simulink model "example_RadiatorAIVtoEN442"  (Simulink 7.6)
settings: Solver=ode45  StartTime=0.0  StopTime=8*3600  RelTol=1e-3
undefined symbols (not defined in the file): A, B, C, Dd
libraries: carnot x9, simulink x1
settings Model: Creator=drhf  LastModifiedBy=drhf
settings CodeAppCC: CustomSymbolStrType=$N$R$M_T

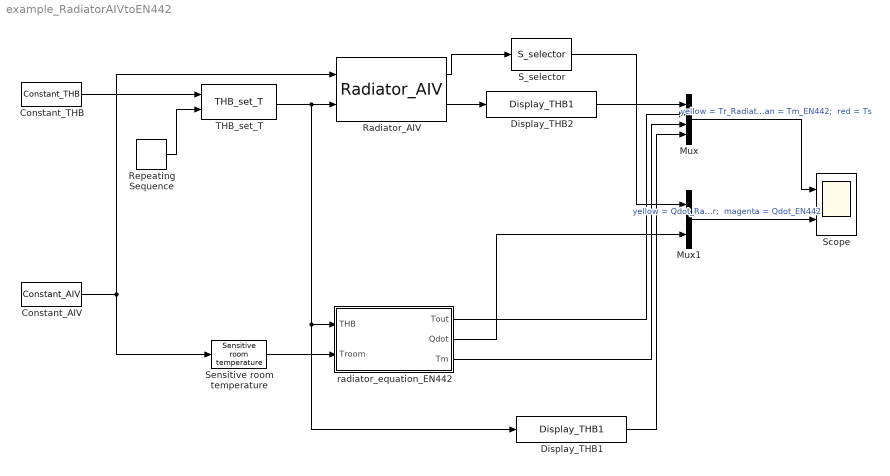
== system example_RadiatorAIVtoEN442 ==
  Constant_AIV : carnot/Source/Ventilation/Constant_AIV  SystemSampleTime=-1  Tsens=20  Tcon=20  Trad=20  mw=0.012  mco=0.01  rhoair=1.2  cpair=1004  pair=100000  nair=0.5
  Constant_THB : carnot/Source/Simple/Constant_THB  SystemSampleTime=-1  t=40  mdot=1000/4182/10  p=1e5  mID=No Pressure Drop  fluid=Water (Constant 20°C)  mix=0  dia=0.02  hgt=0
  Display_THB1 : carnot/Outputs/Display_THB1  SystemSampleTime=-1  t=on  m=off  p=off  id=off  mix=off  d=off
  Display_THB2 : carnot/Outputs/Display_THB1  SystemSampleTime=-1  t=on  m=off  p=off  id=off  mix=off  d=off
  Mux : Mux
  Mux1 : Mux  Inputs=2
  Radiator_AIV : carnot/Source/Heat_Exchanger/Radiator_AIV  SystemSampleTime=-1  pnom=1000  dtnom=50  expo=1.3  mcap=5*4182  ra=0.47  tini=20  lin=10  qua=10
  Repeating Sequence : simulink/Sources/Repeating Sequence  SystemSampleTime=-1  rep_seq_t=[0 2 2.1 4 4.1 6 6.1 8]*3600  rep_seq_y=[45 45 55 55 65 65 75 75]
  S_selector : carnot/Outputs/S_selector  SystemSampleTime=-1  e1=off  e2=off  e3=off  e4=off  e5=on  e6=off  e7=off  e8=off  e9=off  e10=off  e11=off  e12=off  e13=off
  Scope : Scope  NumInputPorts=2
      settings: YMin=-5~-5  YMax=5~5
  Sensitive room temperature : carnot/Outputs/Sensitive room temperature  SystemSampleTime=-1  share_c=47
  THB_set_T : carnot/Source/Simple/THB_set_T  SystemSampleTime=-1
  radiator_equation_EN442 : Subsystem  mask(radiator equation){pnom=1000, dtnom=50, expo=1.3, mcap=10*4200}
      mask prompts: pnom "Qdot_nom: nominal power per in W"; dtnom "Tdiff_nom: nominal temperature difference in K"; expo "radiator exponent (> 0)"; mcap "mass * capacity per unit in J/K"
      mask help:
      | The block calculates the heat transfer of a radiator to a room according to the EN 442 equation:
      | Qdot = Qdot_nom * (Tdiff/Tdiff_nom)^exponent
      | The thermal capacity of the radiator is modeled by a 1-node capacity.
      | mcp*dT/dt = mdot*cp*(Tin-Tnode)-Qdot
  wires:
  Constant_THB/1 -> THB_set_T/1
  THB_set_T/1 -> radiator_equation_EN442/1(THB), Display_THB1/1, Radiator_AIV/2
  Mux/1 -> Scope/1  "yellow = Tr_Radiator;  magenta = Tr_EN442;  cyan = Tm_EN442;  red = Ts"
  Radiator_AIV/2 -> Display_THB2/1
  Repeating Sequence/1 -> THB_set_T/2
  Display_THB2/1 -> Mux/1
  radiator_equation_EN442/1(Tout) -> Mux/2
  S_selector/1 -> Mux1/1
  radiator_equation_EN442/2(Qdot) -> Mux1/2
  Mux1/1 -> Scope/2  "yellow = Qdot_Radiator;  magenta = Qdot_EN442"
  radiator_equation_EN442/3(Tm) -> Mux/3
  Display_THB1/1 -> Mux/4
  Radiator_AIV/1 -> S_selector/1
  Sensitive room temperature/1 -> radiator_equation_EN442/2(Troom)
  Constant_AIV/1 -> Sensitive room temperature/1, Radiator_AIV/1

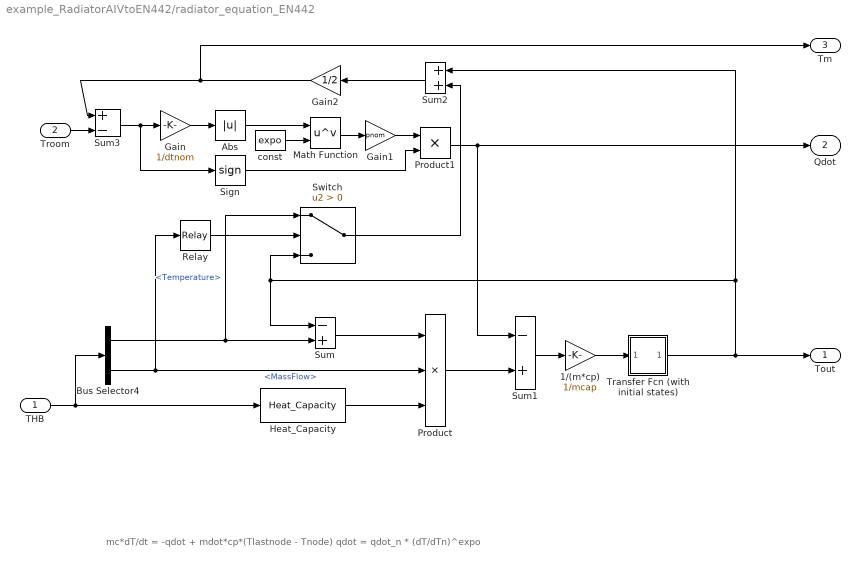
== system example_RadiatorAIVtoEN442/radiator_equation_EN442 ==
  note: mc*dT/dt = -qdot + mdot*cp*(Tlastnode - Tnode)
      |
      | qdot = qdot_n * (dT/dTn)^expo
  THB : Inport
  Troom : Inport  Port=2
  1/(m*cp) : Gain  Gain=1/mcap  SaturateOnIntegerOverflow=on  OutDataTypeStr=Inherit: Same as input  ParamDataTypeStr=Inherit: Same as input
  Abs : Abs  SaturateOnIntegerOverflow=on
  Bus Selector4 : BusSelector  OutputSignals=Temperature,MassFlow
  Gain : Gain  Gain=1/dtnom  SaturateOnIntegerOverflow=on  OutDataTypeStr=Inherit: Same as input  ParamDataTypeStr=Inherit: Same as input
  Gain1 : Gain  Gain=pnom  SaturateOnIntegerOverflow=on  OutDataTypeStr=Inherit: Same as input  ParamDataTypeStr=Inherit: Same as input
  Gain2 : Gain  Gain=1/2  SaturateOnIntegerOverflow=on  OutDataTypeStr=Inherit: Same as input  ParamDataTypeStr=Inherit: Same as input
  Heat_Capacity : carnot/Basic/Material_Properties/Heat_Capacity  SystemSampleTime=-1  VariantObject=CarlibClassic  INPUTARGUMENTS=THB  DEBUGLEVEL=DEBUGLEVEL  MAXTOTALWARNINGS=inf  MAXCONSECUTIVEWARNINGS=inf  WRITETOFILE=0  FILENAME='errors.txt'
  Math Function : Math  Operator=pow  SaturateOnIntegerOverflow=on
  Product : Product  Inputs=3  SaturateOnIntegerOverflow=on  InputSameDT=on  OutDataTypeStr=Inherit: Same as first input
  Product1 : Product  SaturateOnIntegerOverflow=on  InputSameDT=on  OutDataTypeStr=Inherit: Same as first input
  Relay : Relay  OnSwitchValue=1e-5  OffSwitchValue=0
  Sign : Signum
  Sum : Sum  Inputs=-+  SaturateOnIntegerOverflow=on  InputSameDT=on  OutDataTypeStr=Inherit: Same as first input
  Sum1 : Sum  Inputs=-+  SaturateOnIntegerOverflow=on  InputSameDT=on  OutDataTypeStr=Inherit: Same as first input
  Sum2 : Sum  Inputs=2  SaturateOnIntegerOverflow=on  InputSameDT=on  OutDataTypeStr=Inherit: Same as first input
  Sum3 : Sum  Inputs=+-  SaturateOnIntegerOverflow=on  InputSameDT=on  OutDataTypeStr=Inherit: Same as first input
  Switch : Switch  Criteria=u2 > Threshold
  Transfer Fcn (with initial states) : Subsystem  mask(Transfer Function with Initial States){N=[1], D=[1  0], X0=20}
      mask prompts: N "Numerator:"; D "Denominator:"; X0 "Initial conditions:"
      mask help: Vector expressions for numerator, and denominator. Coefficients are in descending powers of s.
      mask init:
      | [A,B,C,Dd]=tf2ss(N,D);if (isempty(X0));[m,n]=size(A);X0=zeros(1,m); end;
      mask Help: Specify the initial states for the transfer function.  The state ordering is determined by the m-file tf2ss.  There is no unique mapping of the states in a transfer function to states in a state-space representation.  However, tf2ss will consistently use the same mapping for a given transfer function.
      mask Display: dpoly(N,D,'s')
  const : Constant  Value=expo
  Tout : Outport
  Qdot : Outport  Port=2
  Tm : Outport  Port=3
  wires:
  Sum2/1 -> Gain2/1
  Gain2/1 -> Sum3/1, Tm/1
  Troom/1 -> Sum3/2
  Sign/1 -> Product1/2
  Sum3/1 -> Sign/1, Gain/1
  Gain1/1 -> Product1/1
  Abs/1 -> Math Function/1
  Gain/1 -> Abs/1
  Math Function/1 -> Gain1/1
  const/1 -> Math Function/2
  Product1/1 -> Qdot/1, Sum1/1
  THB/1 -> Heat_Capacity/1, Bus Selector4/1
  Sum/1 -> Product/1
  Bus Selector4/2 -> Product/2, Relay/1  "<MassFlow>"
  Bus Selector4/1 -> Sum/2, Switch/1  "<Temperature>"
  Heat_Capacity/1 -> Product/3
  Product/1 -> Sum1/2
  Sum1/1 -> 1/(m*cp)/1
  1/(m*cp)/1 -> Transfer Fcn (with initial states)/1(In1)
  Transfer Fcn (with initial states)/1(Out1) -> Sum2/1, Sum/1, Switch/3, Tout/1
  Switch/1 -> Sum2/2
  Relay/1 -> Switch/2

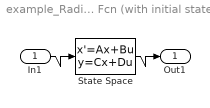
== system example_RadiatorAIVtoEN442/radiator_equation_EN442/Transfer Fcn (with initial states) ==
  In1 : Inport
  State Space : StateSpace  A=A  B=B  C=C  D=Dd  X0=X0
  Out1 : Outport  InitialOutput=0
  wires:
  State Space/1 -> Out1/1
  In1/1 -> State Space/1
